simulink model "sipro_B36_withPWM"  (R2018a)
settings: Solver=ode45  StartTime=0.0  StopTime=10.0  RelTol=1e-3
PreLoadFcn:
  | main;
values from neighbouring files (symbols this model uses):
  C = [1, 0]    [main.m]
  D = 0    [main.m]
  den = [1 0 4]    [main.m]
  E = 0.05    [main.m]
  KD = 0.75    [main.m]
  KI = 2.70    (= 2.7)    [main.m]
  KP = 1.25    [main.m]
  num = [w0*w0*G]    [main.m]
  Tpwm = 0.02    [main.m]
  ts = 0.05    [main.m]
undefined symbols (not defined in the file or in its folder): atilde, btilde
libraries: simulink x3
settings Model: Creator=Sampreet Sarkar  LastModifiedBy=Sampreet Sarkar

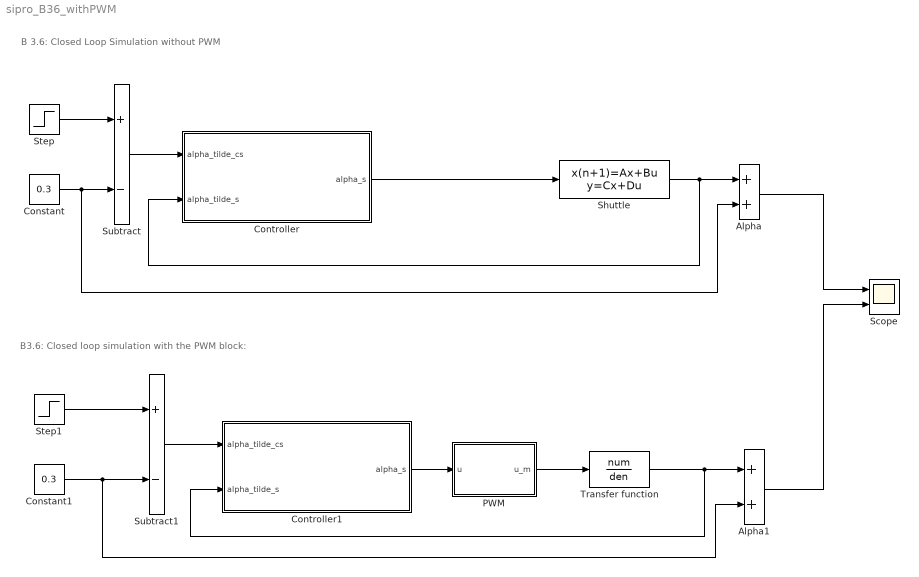
== system sipro_B36_withPWM ==
  note: B3.6: Closed loop simulation with the PWM block:
  note: B 3.6: Closed Loop Simulation without PWM
  Alpha : Sum
  Alpha1 : Sum
  Constant : Constant  Value=0.3
  Constant1 : Constant  Value=0.3
  Controller : Subsystem
  Controller1 : Subsystem
  PWM : Subsystem
  Scope : Scope  NumInputPorts=2
  "Shuttle " : DiscreteStateSpace  A=atilde  B=btilde  C=C  D=D  SampleTime=ts
  Step : Step  Before=0.3  After=0.27  SampleTime=ts
  Step1 : Step  Before=0.3  After=0.27  SampleTime=ts
  Subtract : Sum  Inputs=+-
  Subtract1 : Sum  Inputs=+-
  "Transfer function " : TransferFcn  Numerator=num  Denominator=den
  wires:
  Subtract/1 -> Controller/1(alpha_tilde_cs)
  Constant/1 -> Alpha/2, Subtract/2
  Controller/1(alpha_s) -> "Shuttle "/1
  Step/1 -> Subtract/1
  "Shuttle "/1 -> Alpha/1, Controller/2(alpha_tilde_s)
  PWM/1(u_m) -> "Transfer function "/1
  "Transfer function "/1 -> Controller1/2(alpha_tilde_s), Alpha1/1
  Controller1/1(alpha_s) -> PWM/1(u)
  Step1/1 -> Subtract1/1
  Constant1/1 -> Alpha1/2, Subtract1/2
  Subtract1/1 -> Controller1/1(alpha_tilde_cs)
  Alpha/1 -> Scope/1
  Alpha1/1 -> Scope/2

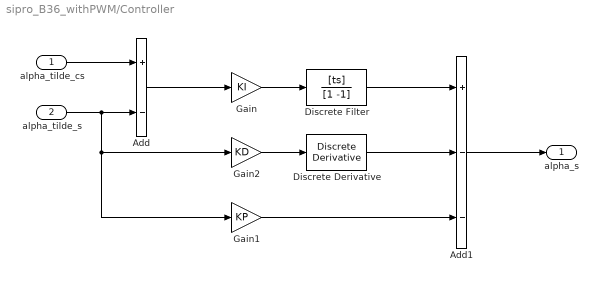
== system sipro_B36_withPWM/Controller ==
  alpha_tilde_cs : Inport
  alpha_tilde_s : Inport  Port=2
  Add : Sum  Inputs=+-
  Add1 : Sum  Inputs=+--
  Discrete Derivative : simulink/Discrete/Discrete Derivative  gainval=1.0  ICPrevScaledInput=0.0  OutMin=[]  OutMax=[]  OutDataType=fixdt(1, 16)  OutScaling=2^-10  DoSatur=off
  Discrete Filter : DiscreteFilter  Numerator=[ts]  Denominator=[1 -1]
  Gain : Gain  Gain=KI
  Gain1 : Gain  Gain=KP
  Gain2 : Gain  Gain=KD
  alpha_s : Outport
  wires:
  Gain2/1 -> Discrete Derivative/1
  Discrete Filter/1 -> Add1/1
  Add/1 -> Gain/1
  Gain/1 -> Discrete Filter/1
  alpha_tilde_s/1 -> Gain1/1, Gain2/1, Add/2
  Discrete Derivative/1 -> Add1/2
  alpha_tilde_cs/1 -> Add/1
  Gain1/1 -> Add1/3
  Add1/1 -> alpha_s/1

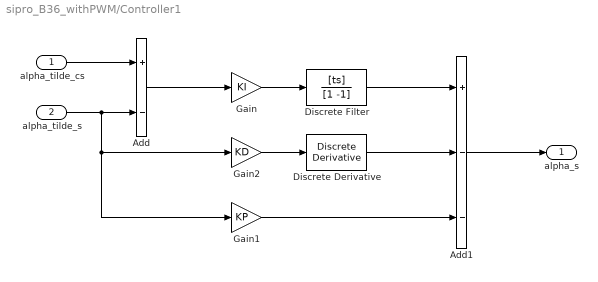
== system sipro_B36_withPWM/Controller1 ==
  alpha_tilde_cs : Inport
  alpha_tilde_s : Inport  Port=2
  Add : Sum  Inputs=+-
  Add1 : Sum  Inputs=+--
  Discrete Derivative : simulink/Discrete/Discrete Derivative  gainval=1.0  ICPrevScaledInput=0.0  OutMin=[]  OutMax=[]  OutDataType=fixdt(1, 16)  OutScaling=2^-10  DoSatur=off
  Discrete Filter : DiscreteFilter  Numerator=[ts]  Denominator=[1 -1]
  Gain : Gain  Gain=KI
  Gain1 : Gain  Gain=KP
  Gain2 : Gain  Gain=KD
  alpha_s : Outport
  wires:
  Gain2/1 -> Discrete Derivative/1
  Discrete Filter/1 -> Add1/1
  Add/1 -> Gain/1
  Gain/1 -> Discrete Filter/1
  alpha_tilde_s/1 -> Gain1/1, Gain2/1, Add/2
  Discrete Derivative/1 -> Add1/2
  alpha_tilde_cs/1 -> Add/1
  Gain1/1 -> Add1/3
  Add1/1 -> alpha_s/1

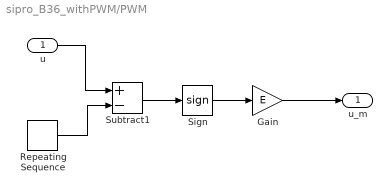
== system sipro_B36_withPWM/PWM ==
  u : Inport
  Gain : Gain  Gain=E
  Repeating Sequence : simulink/Sources/Repeating Sequence  rep_seq_t=[0: (Tpwm/2): (Tpwm)]  rep_seq_y=[-E +E -E]
  Sign : Signum
  Subtract1 : Sum  Inputs=+-
  u_m : Outport
  wires:
  Repeating Sequence/1 -> Subtract1/2
  Gain/1 -> u_m/1
  Subtract1/1 -> Sign/1
  Sign/1 -> Gain/1
  u/1 -> Subtract1/1
